simulink model "simulink fm"  (R2025a)
settings: Solver=VariableStepAuto  StartTime=0.0  StopTime=10.0  RelTol=1e-3
settings Model: Creator=hp  LastModifiedBy=hp

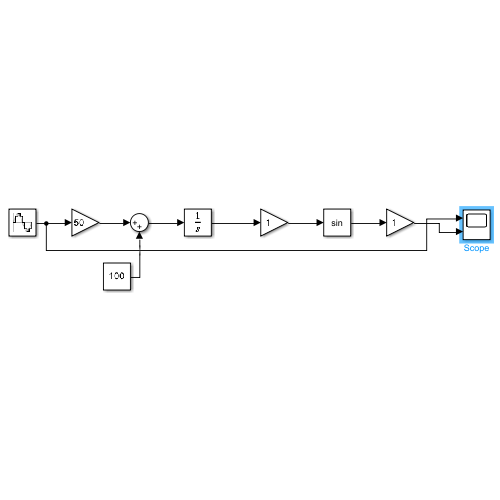
[thumbnail: Simulink's stored preview of the top-level diagram]
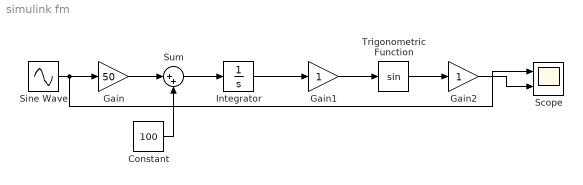
== system simulink fm ==
  Constant : Constant  Value=100
  Gain : Gain  Gain=50
  Gain1 : Gain
  Gain2 : Gain
  Integrator : Integrator
  Scope : Scope  NumInputPorts=2
      settings: ActiveDisplayYMinimum=-1.2499999999999871  ActiveDisplayYMaximum=1.2499999999999944
  Sine Wave : Sin  Frequency=2*pi  SampleTime=1/1000
  Sum : Sum  Inputs=|++
  Trigonometric Function : Trigonometry
  wires:
  Sine Wave/1 -> Scope/1, Gain/1
  Gain/1 -> Sum/1
  Constant/1 -> Sum/2
  Sum/1 -> Integrator/1
  Integrator/1 -> Gain1/1
  Gain1/1 -> Trigonometric Function/1
  Trigonometric Function/1 -> Gain2/1
  Gain2/1 -> Scope/2
